simulink model "CB_OL_Harness"  (R2015b)
settings: Solver=FixedStepAuto  StartTime=0.0  StopTime=sim_time  FixedStep=0.01  RelTol=1e-3
libraries: simulink x1
settings Model: Creator=favv5g  LastModifiedBy=favv5g
settings HardwareCC: ProdBitPerPointer=32  ProdLargestAtomicInteger=Long  ProdLargestAtomicFloat=Double  ProdEndianess=BigEndian  ProdWordSize=32  ProdHWDeviceType=Freescale->32-bit PowerPC

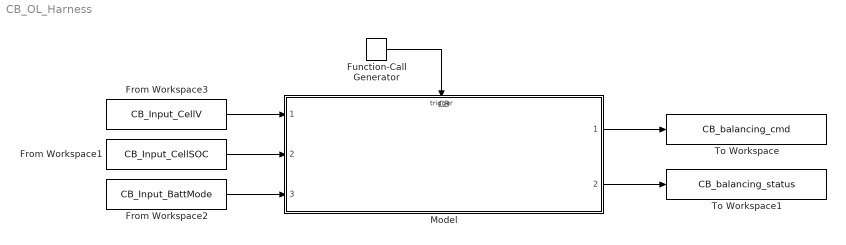
== system CB_OL_Harness ==
  From Workspace1 : FromWorkspace  VariableName=CB_Input_CellSOC
  From Workspace2 : FromWorkspace  VariableName=CB_Input_BattMode
  From Workspace3 : FromWorkspace  VariableName=CB_Input_CellV
  Function-Call Generator : simulink/Ports & Subsystems/Function-Call Generator  sample_time=0.01  numberOfIterations=1
  Model : ModelReference  ModelNameDialog=CB.slx  SimulationMode=Normal  ModelReferenceVersion=1.20  CopyOfModelName=CB.slx  TriggerPortName=Trigger  TriggerPortTriggerType=function-call  TriggerPortStatesWhenEnabling=held
  To Workspace : ToWorkspace  VariableName=CB_balancing_cmd  SaveFormat=Timeseries  SampleTime=-1
  To Workspace1 : ToWorkspace  VariableName=CB_balancing_status  SaveFormat=Timeseries  SampleTime=-1
  wires:
  From Workspace3/1 -> Model/1
  From Workspace1/1 -> Model/2
  From Workspace2/1 -> Model/3
  Model/1 -> To Workspace/1
  Model/2 -> To Workspace1/1
  Function-Call Generator/1 -> Model/Trigger
